simulink model "SDRE_MPTA_SDRE"  (R2024a)
settings: Solver=ode23tb  StartTime=0  StopTime=1  RelTol=1e-3
values from neighbouring files (symbols this model uses):
  B = 0.002277    [initial_value.m]
  J = 0.00782    [initial_value.m]
  Lambda_m = 0.30175    [initial_value.m]
  Ld = 18e-3    (= 0.018)    [initial_value.m]
  Ldq = Ld - Lq    [inital.m]
  Lq = 32e-3    (= 0.032)    [initial_value.m]
  Polepairs = 3    [initial_value.m]
  rate1 = 3    [inital.m]
  rate2 = 1    [inital.m]
  Rs = 2.5    [initial_value.m]
  timestep = 1e-5    (= 1e-05)    [inital.m]
  V = [V_11 V_12;V_21 V_22]    [Create_MVG.m]
undefined symbols (not defined in the file or in its folder): rate
libraries: spsControlledVoltageSourceLib x12, mcbcontrolslib x4, spsGroundLib x4, spsPermanentMagnetSynchronousMachineLib x2, sps_lib x1
(part 2 of 2)

== system SDRE_MPTA_SDRE/nomal2/toq to voltageABC/If Action Subsystem2 ==
  In1 : Inport
  Action Port : ActionPort  ActionPortLabel=else
  Out1 : Outport
  wires:
  In1/1 -> Out1/1

== system SDRE_MPTA_SDRE/nomal2/toq to voltageABC/If Action Subsystem3 ==
  In1 : Inport
  Action Port : ActionPort  ActionPortLabel=if(u1 < 1e-10)
  Out1 : Outport
  wires:
  In1/1 -> Out1/1

== system SDRE_MPTA_SDRE/nomal2/toq to voltageABC/Subsystem ==
  In1 : Inport
  In2 : Inport  Port=2
  In3 : Inport  Port=3
  Add : Sum
  Constant : Constant  Value=3*Polepairs/2
  Constant1 : Constant  Value=Lambda_m
  Gain : Gain  Gain=Ldq
  Product : Product
  Product1 : Product
  Product2 : Product
  Out1 : Outport
  wires:
  Product1/1 -> Add/2
  Product2/1 -> Gain/1
  Product/1 -> Out1/1
  Constant/1 -> Product/2
  In3/1 -> Product2/1
  Add/1 -> Product/1
  Gain/1 -> Add/1
  Constant1/1 -> Product1/2
  In1/1 -> Product2/2
  In2/1 -> Product1/1

== system SDRE_MPTA_SDRE/nomal2/toq to voltageABC6/Inverse Clarke Transform ==
  note: Inverse Clarke Transform
  note: Converts direct axis (alpha) component and the quadrature axis (beta) component to balanced three-phase quantities
      | The alpha and beta components are dependent on time and speed.
  Alpha : Inport
  Beta : Inport  Port=2
  Add : Sum  Inputs=-+  OutDataTypeStr=Inherit: Same as first input
  Add1 : Sum  Inputs=--  OutDataTypeStr=Inherit: Same as first input
  Gain : Gain  Gain=1/2
  Gain1 : Gain  Gain=sqrt(3)/2
  Mux : Mux  Inputs=3
  ABC : Outport  VectorParamsAs1DForOutWhenUnconnected=off
  wires:
  Beta/1 -> Gain1/1
  Mux/1 -> ABC/1
  Alpha/1 -> Mux/1, Gain/1
  Add1/1 -> Mux/3
  Gain1/1 -> Add1/2, Add/2
  Gain/1 -> Add1/1, Add/1
  Add/1 -> Mux/2

== system SDRE_MPTA_SDRE/nomal2/toq to voltageABC6/Inverse Park Transform ==
  note: Converts orthogonal rotating reference frame (dq) to two-phase orthogonal stationary reference frame (alpha, beta)
  note: Inverse Park Transform
  D : Inport
  Q : Inport  Port=2
  Sin_Coefficient : Inport  Port=3
  Cos_Coefficient : Inport  Port=4
  Add1 : Sum  Inputs=+-  OutDataTypeStr=Inherit: Same as first input
  Add2 : Sum  OutDataTypeStr=Inherit: Same as first input
  Cos_Coefficient_1 : InportShadow  Port=4
  Product{1..4} (4 alike) : Product  RndMeth=Simplest
  Sin_Coefficient_1 : InportShadow  Port=3
  Alpha : Outport  VectorParamsAs1DForOutWhenUnconnected=off
  Beta : Outport  Port=2  VectorParamsAs1DForOutWhenUnconnected=off
  wires:
  Sin_Coefficient_1/1 -> Product3/2
  Product2/1 -> Add1/2
  Cos_Coefficient_1/1 -> Product4/2
  Add2/1 -> Beta/1
  Product3/1 -> Add2/1
  Add1/1 -> Alpha/1
  Product1/1 -> Add1/1
  Product4/1 -> Add2/2
  Sin_Coefficient/1 -> Product2/2
  D/1 -> Product3/1, Product1/1
  Q/1 -> Product2/1, Product4/1
  Cos_Coefficient/1 -> Product1/2

== system SDRE_MPTA_SDRE/nomal2/toq to voltageABC6/Subsystem ==
  In1 : Inport
  Bus Selector : BusSelector  OutputSignals=Rotor speed wm (rad/s),Stator current is_d (A),Stator current is_q (A)
  Divide5 : Product  Commented=on  Inputs=*/
  Gain1 : Gain  Gain=Polepairs
  Rate_Transition2 : RateTransition  Integrity=off  Deterministic=off
  Rate_Transition3 : RateTransition  Integrity=off  Deterministic=off
  Rate_Transition4 : RateTransition  Integrity=off  Deterministic=off
  Scope : Scope
  Subsystem : Subsystem
  rad/s to rpm : Gain  Gain=60/(2*pi)
  Out1 : Outport
  Out2 : Outport  Port=2
  Out3 : Outport  Port=3
  wires:
  Gain1/1 -> rad/s to rpm/1
  rad/s to rpm/1 -> Rate_Transition2/1
  Rate_Transition4/1 -> Subsystem/2(In2), Subsystem/3(In3), Out3/1
  Bus Selector/1 -> Gain1/1  "<Rotor speed wm (rad/s)>"
  Bus Selector/3 -> Rate_Transition4/1  "<Stator current is_q (A)>"
  Bus Selector/2 -> Rate_Transition3/1  "<Stator current is_d (A)>"
  In1/1 -> Bus Selector/1
  Rate_Transition3/1 -> Subsystem/1(In1), Out1/1
  Rate_Transition2/1 -> Out2/1
  Subsystem/1(Out1) -> Scope/1

== system SDRE_MPTA_SDRE/nomal2/toq to voltageABC6/Subsystem1 ==
  In1 : Inport
  Rate_Transition1 : RateTransition  Integrity=off
  Out1 : Outport  VectorParamsAs1DForOutWhenUnconnected=off
  wires:
  In1/1 -> Rate_Transition1/1
  Rate_Transition1/1 -> Out1/1

== system SDRE_MPTA_SDRE/nomal2/toq to voltageABC6/Subsystem2 ==
  In1 : Inport
  In2 : Inport  Port=2
  In3 : Inport  Port=3
  Derivative : Derivative
  Derivative1 : Derivative
  Gain : Gain  Gain=Polepairs
  ras/s to rev/min : Gain  Gain=60/(2*pi)
  Out1 : Outport
  Out2 : Outport  Port=2
  Out3 : Outport  Port=3
  Out4 : Outport  Port=4
  Out5 : Outport  Port=5
  wires:
  Gain/1 -> ras/s to rev/min/1
  In2/1 -> Derivative/1, Out2/1
  ras/s to rev/min/1 -> Out1/1
  In3/1 -> Derivative1/1, Out3/1
  In1/1 -> Gain/1
  Derivative/1 -> Out4/1
  Derivative1/1 -> Out5/1

== system SDRE_MPTA_SDRE/nomal2/toq to voltageABC6/ideal_voltage_source ==
  note: PWM Peripheral And Inverter
  Vabc : Inport
  Controlled_Voltage_Source1 : spsControlledVoltageSourceLib/Controlled Voltage Source  Initialize=off  Source_Type=DC  Amplitude=12  Phase=0  Frequency=0  Measurements=Voltage
  Controlled_Voltage_Source2 : spsControlledVoltageSourceLib/Controlled Voltage Source  Initialize=off  Source_Type=DC  Amplitude=12  Phase=0  Frequency=0  Measurements=Voltage
  Controlled_Voltage_Source3 : spsControlledVoltageSourceLib/Controlled Voltage Source  Initialize=off  Source_Type=DC  Amplitude=12  Phase=0  Frequency=0  Measurements=Voltage
  Ground2 : spsGroundLib/Ground  LConnTagsString=a
  Scope : Scope  NumInputPorts=3
  Selector3 : Selector  InputPortWidth=3  IndexOptions=Index vector (dialog)  Indices=[1]  OutputSizes=1
  Selector4 : Selector  InputPortWidth=3  IndexOptions=Index vector (dialog)  Indices=2  OutputSizes=1
  Selector5 : Selector  InputPortWidth=3  IndexOptions=Index vector (dialog)  Indices=3  OutputSizes=1
  A : PMIOPort  Tag=PMCPort  Side=Right
  B : PMIOPort  Tag=PMCPort  Port=2  Side=Right
  C : PMIOPort  Tag=PMCPort  Port=3  Side=Right
  wires:
  Vabc/1 -> Selector4/1, Selector5/1, Selector3/1
  Selector5/1 -> Scope/3, Controlled_Voltage_Source3/1
  Selector4/1 -> Scope/2, Controlled_Voltage_Source2/1
  Selector3/1 -> Scope/1, Controlled_Voltage_Source1/1
  connections:
  C/RConn1 -- Controlled_Voltage_Source3/RConn1
  B/RConn1 -- Controlled_Voltage_Source2/RConn1
  A/RConn1 -- Controlled_Voltage_Source1/RConn1
  Controlled_Voltage_Source3/LConn1 -- Controlled_Voltage_Source1/LConn1 -- Controlled_Voltage_Source2/LConn1 -- Ground2/LConn1

== system SDRE_MPTA_SDRE/nomal2/toq to voltageABC6/ideal_voltage_source1 ==
  note: PWM Peripheral And Inverter
  Vabc : Inport
  Controlled_Voltage_Source1 : spsControlledVoltageSourceLib/Controlled Voltage Source  Initialize=off  Source_Type=DC  Amplitude=12  Phase=0  Frequency=0  Measurements=None
  Controlled_Voltage_Source2 : spsControlledVoltageSourceLib/Controlled Voltage Source  Initialize=off  Source_Type=DC  Amplitude=12  Phase=0  Frequency=0  Measurements=None
  Controlled_Voltage_Source3 : spsControlledVoltageSourceLib/Controlled Voltage Source  Initialize=off  Source_Type=DC  Amplitude=12  Phase=0  Frequency=0  Measurements=None
  Ground2 : spsGroundLib/Ground  LConnTagsString=a
  Selector3 : Selector  InputPortWidth=3  IndexOptions=Index vector (dialog)  Indices=[1]  OutputSizes=1
  Selector4 : Selector  InputPortWidth=3  IndexOptions=Index vector (dialog)  Indices=2  OutputSizes=1
  Selector5 : Selector  InputPortWidth=3  IndexOptions=Index vector (dialog)  Indices=3  OutputSizes=1
  A : PMIOPort  Tag=PMCPort  Side=Right
  B : PMIOPort  Tag=PMCPort  Port=2  Side=Right
  C : PMIOPort  Tag=PMCPort  Port=3  Side=Right
  wires:
  Vabc/1 -> Selector4/1, Selector5/1, Selector3/1
  Selector5/1 -> Controlled_Voltage_Source3/1
  Selector4/1 -> Controlled_Voltage_Source2/1
  Selector3/1 -> Controlled_Voltage_Source1/1
  connections:
  C/RConn1 -- Controlled_Voltage_Source3/RConn1
  B/RConn1 -- Controlled_Voltage_Source2/RConn1
  A/RConn1 -- Controlled_Voltage_Source1/RConn1
  Controlled_Voltage_Source3/LConn1 -- Controlled_Voltage_Source1/LConn1 -- Controlled_Voltage_Source2/LConn1 -- Ground2/LConn1

== system SDRE_MPTA_SDRE/nomal1/toq to voltageABC6/Subsystem/Subsystem ==
  In1 : Inport
  In2 : Inport  Port=2
  In3 : Inport  Port=3
  Add : Sum
  Constant : Constant  Value=3*Polepairs/2
  Constant1 : Constant  Value=Lambda_m
  Gain : Gain  Gain=Ldq
  Product : Product
  Product1 : Product
  Product2 : Product
  Out1 : Outport
  wires:
  Product1/1 -> Add/2
  Product2/1 -> Gain/1
  Product/1 -> Out1/1
  Constant/1 -> Product/2
  In3/1 -> Product2/1
  Add/1 -> Product/1
  Gain/1 -> Add/1
  Constant1/1 -> Product1/2
  In1/1 -> Product2/2
  In2/1 -> Product1/1

== system SDRE_MPTA_SDRE/nomal2/toq to voltageABC6/Subsystem/Subsystem ==
  In1 : Inport
  In2 : Inport  Port=2
  In3 : Inport  Port=3
  Add : Sum
  Constant : Constant  Value=3*Polepairs/2
  Constant1 : Constant  Value=Lambda_m
  Gain : Gain  Gain=Ldq
  Product : Product
  Product1 : Product
  Product2 : Product
  Out1 : Outport
  wires:
  Product1/1 -> Add/2
  Product2/1 -> Gain/1
  Product/1 -> Out1/1
  Constant/1 -> Product/2
  In3/1 -> Product2/1
  Add/1 -> Product/1
  Gain/1 -> Add/1
  Constant1/1 -> Product1/2
  In1/1 -> Product2/2
  In2/1 -> Product1/1

== matlab function SDRE_MPTA_SDRE/target path input1/Subsystem1/Path function ==
  data: time input; Place output; Velocity output; Acc output
function [Place,Velocity,Acc] = fcn(time)



Place = (time^3)/4 *pi;
Velocity = 3/4 * time^2 *pi*10;
Acc = 3/2 * time * pi*10^2;


end

== matlab function SDRE_MPTA_SDRE/target path input1/Subsystem2/Path function ==
  data: time input; Place output; Velocity output; Acc output
function [Place,Velocity,Acc] = fcn(time)



% Place = time^3 /4 *pi;
% Velocity = 3/4 * time^2 *pi;
% Acc = 3/2 * time * pi;

Place = time^3 /4 *pi;
Velocity = 3/4 * time^2 *pi*10;
Acc = 3/2 * time * pi*10^2;

end

== matlab function SDRE_MPTA_SDRE/nomal2/toq to voltageABC6/MATLAB Function1 ==
  data: velo_fb input; id_fb input; iq_fb input; velo_ref input; id_ref input; iq_ref input; ud output; uq output; ud1 output; uq1 output; id_dot input; iq_dot input; ud2 output; uq2 output; velo_error output; id_error output; iq_error output
function [ud,uq,ud1,uq1,ud2,uq2,velo_error,id_error,iq_error] = SDRE_motor(velo_fb,id_fb,iq_fb,velo_ref,id_ref,iq_ref,id_dot,iq_dot)

ud = zeros(1, 1, 'double');
uq = zeros(1, 1, 'double');

%change data from [1*1] to singal input
Q = zeros(3, 3, 'double');

if isempty(id_dot)
    id_dot=0;
    iq_dot=0;
end


% velo_error   = 0;
% id_error     = 0;
% iq_error     = 0;

velo_error   = velo_fb   - velo_ref;
id_error     = id_fb     - id_ref;
iq_error     = iq_fb     - iq_ref;

if isempty(iq_error)
    velo_error=0;
    id_error=0;
    iq_error =0;
end

error = [velo_error iq_error id_error];

[Ld,Lq,Rs,Lambda_m,Polepairs,J,B]  = initial_value;
Ldq = Ld-Lq;

% A11 = -B/J; A12 = 3*Polepairs^2 *Lambda_m/(8*J); A13 = 3*Polepairs^2 *Ldq*iq_error/(8*J);
% A21 = -Lambda_m/(Lq) - Ld*id_error/(2*Lq); A22 = -Rs/Lq; A23 = - Ld*velo_error/(2*Lq);
% A31 = Lq*iq_error/(2*Ld); A32 =Lq*velo_error/(2*Ld); A33 = -Rs/Ld;

A11 = -B/J; A12 = 3*Polepairs^2 *Lambda_m/(4*J); A13 = 3*Polepairs^2 *Ldq*iq_error/(4*J);
A21 = -Lambda_m/(Lq) - Ld*id_error/(Lq); A22 = -Rs/Lq; A23 = 0;
A31 = Lq*iq_error/(Ld); A32 =0; A33 = -Rs/Ld;

B11 = 0;B12 =0;
B21=1/Lq;B22=0;
B31=0;B32=1/Ld;


A = [A11 A12 A13 ;
     A21 A22 A23 ;
     A31 A32 A33];

B = [B11 B12;
     B21 B22;
     B31 B32];


rate = sqrt(iq_error^2 + id_error^2);

Q=diag([800 1+exp(-rate) 100+exp(-rate)]);
R=diag([1 1]);

[P_ss_care,~]=SDA_CARE(A,B,Q,R);


% ucq = Rs*iq_ref + Lq*iq_dot + velo_ref*(Ld*id_ref+Lambda_m);
% ucd = Rs*id_ref + Ld*id_dot - velo_ref*Lq*iq_ref;


ucq = Rs*iq_ref + Lambda_m*velo_ref + Lq*iq_dot + Ld*id_error*velo_ref + Ld*velo_fb*id_ref;
ucd = Rs*id_ref + Ld*id_dot - Lq*iq_error*velo_ref - Lq*velo_fb*iq_ref;
if ucq > 1e5
    ucq =0;
end

if ucd > 1e5
    ucd =0;
end

u_redeem = -inv(R)*B'*P_ss_care*error';

% uq =  ucq ;
% ud =  ucd ;

uq =  ucq + u_redeem(1) ;
ud =  ucd + u_redeem(2) ;

ud1 = ucd ;
uq1 = ucq;

ud2 = u_redeem(2) ;
uq2 = u_redeem(1) ;


ud = (reshape(ud, 1, 1));
uq = (reshape(uq, 1, 1));


end

== matlab function SDRE_MPTA_SDRE/nomal1/toq to voltageABC6/MATLAB Function1 ==
  data: velo_fb input; id_fb input; iq_fb input; velo_ref input; id_ref input; iq_ref input; ud output; uq output; ud1 output; uq1 output; id_dot input; iq_dot input; ud2 output; uq2 output; velo_error output; id_error output; iq_error output
function [ud,uq,ud1,uq1,ud2,uq2,velo_error,id_error,iq_error] = SDRE_motor(velo_fb,id_fb,iq_fb,velo_ref,id_ref,iq_ref,id_dot,iq_dot)

ud = zeros(1, 1, 'double');
uq = zeros(1, 1, 'double');

%change data from [1*1] to singal input
Q = zeros(3, 3, 'double');

if isempty(id_dot)
    id_dot=0;
    iq_dot=0;
end


% velo_error   = 0;
% id_error     = 0;
% iq_error     = 0;

velo_error   = velo_fb   - velo_ref;
id_error     = id_fb     - id_ref;
iq_error     = iq_fb     - iq_ref;

if isempty(iq_error)
    velo_error=0;
    id_error=0;
    iq_error =0;
end

error = [velo_error iq_error id_error];

[Ld,Lq,Rs,Lambda_m,Polepairs,J,B]  = initial_value;
Ldq = Ld-Lq;

% A11 = -B/J; A12 = 3*Polepairs^2 *Lambda_m/(8*J); A13 = 3*Polepairs^2 *Ldq*iq_error/(8*J);
% A21 = -Lambda_m/(Lq) - Ld*id_error/(2*Lq); A22 = -Rs/Lq; A23 = - Ld*velo_error/(2*Lq);
% A31 = Lq*iq_error/(2*Ld); A32 =Lq*velo_error/(2*Ld); A33 = -Rs/Ld;

A11 = -B/J; A12 = 3*Polepairs^2 *Lambda_m/(4*J); A13 = 3*Polepairs^2 *Ldq*iq_error/(4*J);
A21 = -Lambda_m/(Lq) - Ld*id_error/(Lq); A22 = -Rs/Lq; A23 = 0;
A31 = Lq*iq_error/(Ld); A32 =0; A33 = -Rs/Ld;

B11 = 0;B12 =0;
B21=1/Lq;B22=0;
B31=0;B32=1/Ld;


A = [A11 A12 A13 ;
     A21 A22 A23 ;
     A31 A32 A33];

B = [B11 B12;
     B21 B22;
     B31 B32];


rate = sqrt(iq_error^2 + id_error^2);

Q=diag([800 1+exp(-rate) 100+exp(-rate)]);
R=diag([1 1]);

[P_ss_care,~]=SDA_CARE(A,B,Q,R);


% ucq = Rs*iq_ref + Lq*iq_dot + velo_ref*(Ld*id_ref+Lambda_m);
% ucd = Rs*id_ref + Ld*id_dot - velo_ref*Lq*iq_ref;


ucq = Rs*iq_ref + Lambda_m*velo_ref + Lq*iq_dot + Ld*id_error*velo_ref + Ld*velo_fb*id_ref;
ucd = Rs*id_ref + Ld*id_dot - Lq*iq_error*velo_ref - Lq*velo_fb*iq_ref;
if ucq > 1e5
    ucq =0;
end

if ucd > 1e5
    ucd =0;
end

u_redeem = -inv(R)*B'*P_ss_care*error';

% uq =  ucq ;
% ud =  ucd ;

uq =  ucq + u_redeem(1) ;
ud =  ucd + u_redeem(2) ;

ud1 = ucd ;
uq1 = ucq;

ud2 = u_redeem(2) ;
uq2 = u_redeem(1) ;


ud = (reshape(ud, 1, 1));
uq = (reshape(uq, 1, 1));


end

== matlab function SDRE_MPTA_SDRE/SDRE1 ==
  data: output_u1 output; Velocity1_ref output; T_load_1 output; Theta1_fb input; Velocity1_fb input; Acc1_fb input; Theta1_ref input; Theta2_ref input; Velocity1_ref input; Velocity2_ref input; Acc1_ref input; Acc2_ref input; display1 output; display2 output; output_u2 output; Velocity2_ref output; T_load_2 output; Theta2_fb input; Velocity2_fb input; Acc2_fb input; time input
function [output_u1,Velocity1_ref,T_load_1,display1,display2,output_u2,Velocity2_ref,T_load_2] = Motor_state(Theta1_fb,Velocity1_fb,Acc1_fb,Theta1_ref,Theta2_ref,Velocity1_ref,Velocity2_ref,Acc1_ref,Acc2_ref, Theta2_fb,  Velocity2_fb,Acc2_fb,time)
    %change data from [1*1] to singal input
    Acc2_ref = reshape(Acc2_ref, 1, []);

    Theta1_error =Theta1_fb - Theta1_ref;
    Velocity1_error = Velocity1_fb - Velocity1_ref;
    Acc1_error = Acc1_ref - Acc1_fb;

    Theta2_error = Theta2_fb - Theta2_ref;    
    Velocity2_error = Velocity2_fb - Velocity2_ref;
    Acc2_error = Acc2_ref - Acc2_fb;

    % Theta1_error = 0;
    % Velocity1_error = 0;
    % Acc1_error = 0;
    % Theta2_error = 0;       
    % Velocity2_error = 0;  
    % Acc2_error =0;
    
    Acc_ref = [Acc1_ref;Acc2_ref];
    Velo_ref = [Velocity1_ref;Velocity2_ref];
    Theta_ref = [Theta1_ref;Theta2_ref];
    error_robot = [Theta1_error Theta2_error Velocity1_error Velocity2_error 0];

    Q=diag([10 10 1000 1000 0]);
    R=diag([1 1]);

    zeta = 10*exp(-5*time);

    [M_fb,V_fb,G_sd_fb]=Create_MVG(Theta1_fb,Theta2_fb,Velocity1_fb,Velocity2_fb);
    [M_ref,V_ref,G_sd_ref]=Create_MVG(Theta1_ref,Theta2_ref,Velocity1_ref,Velocity2_ref);
    gf = M_fb*Acc_ref - M_ref*Acc_ref + V_fb*Velo_ref - V_ref*Velo_ref + G_sd_fb*Theta_ref - G_sd_ref*Theta_ref;
    A11 = zeros(2);
    A12 = eye(2);
    A13 = [0;0];
    A21 = -(M_fb)\G_sd_fb;
    A22 = -(M_fb)\V_fb;
    A23 = -((M_fb)\gf)/zeta;
    A31 = [0 0];
    A32 = [0 0];
    A33 = -5;
    A = [A11 A12 A13;A21 A22 A23;A31 A32 A33];
    B1 = zeros(2);
    B2 = inv(M_fb);
    B = [B1;B2;0 0];
    [P_ss_care,~]=SDA_CARE(A,B,Q,R);
    
    u1 = -inv(R)*B'*P_ss_care*error_robot';
    u_f1_1 = M_ref*[Acc1_ref Acc2_ref]';
    u_f1_2 = V_ref*[Velocity1_ref Velocity2_ref]';
    u_f1_3 = G_sd_ref*[Theta1_ref Theta2_ref]';
    u_f1 =  u_f1_1 + u_f1_2 + u_f1_3;

    output_u1 = u1(1) + u_f1(1);
    output_u2 = u1(2) + u_f1(2);

    [Ld,Lq,Rs,Lambda_m,Polepairs,J,B] = initial_value;
    ul_f1_1 = M_fb*[Acc1_fb Acc2_fb]';
    ul_f1_2 = V_fb*[Velocity1_fb Velocity2_fb]';
    ul_f1_3 = G_sd_fb*[Theta1_fb Theta2_fb]';
    ul_f1 =  ul_f1_1 + ul_f1_2 + ul_f1_3;
    % T_load_1 = ul_f1(1) ;
    % T_load_2 = ul_f1(2) ;
    display1 = ul_f1(1) ;
    display2 = ul_f1(2) ;   
    % 
    T_load_1 = u_f1(1) - J*Acc1_fb - B*Velocity1_fb - J*Acc1_error - B*Velocity1_error;
    T_load_2 = u_f1(2) - J*Acc2_fb - B*Velocity2_fb - J*Acc2_error - B*Velocity2_error;


    % output_u1 = (u1(1) + u_f1(1)) - T_load_1;
    % output_u2 = (u1(2) + u_f1(2)) - T_load_2 ;

    
end
